simulink model "furuta_rl_balance"  (R2025a)
settings: Solver=VariableStepAuto  StartTime=0.0  StopTime=50  RelTol=1e-3
libraries: rllib x1
settings Model: Creator=deng_zhiwen  LastModifiedBy=deng_zhiwen

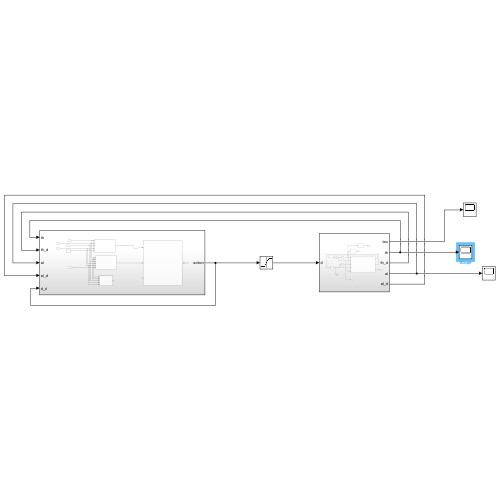
[thumbnail: Simulink's stored preview of the top-level diagram]
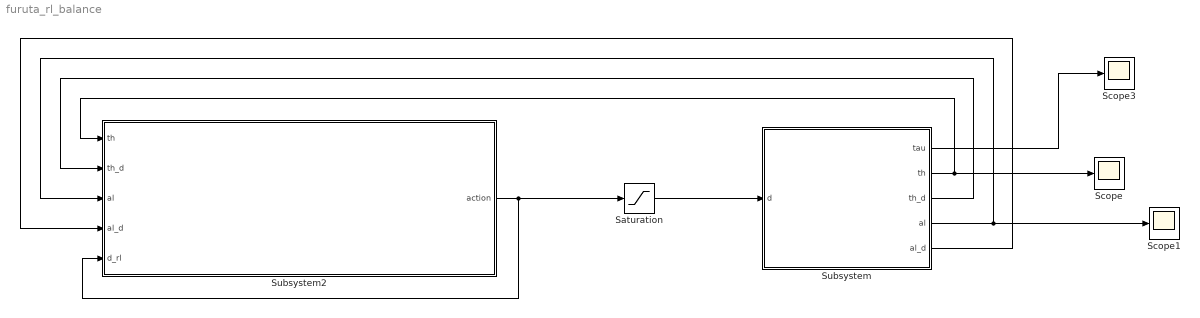
== system furuta_rl_balance ==
  Saturation : Saturate  UpperLimit=1  LowerLimit=-1
  Scope : Scope
      settings: ActiveDisplayYMinimum=-7.2129032176721157  ActiveDisplayYMaximum=4.9641994886210785
  Scope1 : Scope
      settings: ActiveDisplayYMinimum=-7.2858875046268059  ActiveDisplayYMaximum=4.4859787074197675
  Scope3 : Scope
      settings: ActiveDisplayYMinimum=-1  ActiveDisplayYMaximum=1  DataLoggingVariableName=ScopeData3
  Subsystem : Subsystem
  Subsystem2 : Subsystem
  wires:
  Subsystem/2(th) -> Scope/1, Subsystem2/1(th)
  Subsystem/3(th_d) -> Subsystem2/2(th_d)
  Subsystem/4(al) -> Scope1/1, Subsystem2/3(al)
  Subsystem/5(al_d) -> Subsystem2/4(al_d)
  Subsystem2/1(action) -> Saturation/1, Subsystem2/5(d_rl)
  Saturation/1 -> Subsystem/1(d)
  Subsystem/1(tau) -> Scope3/1

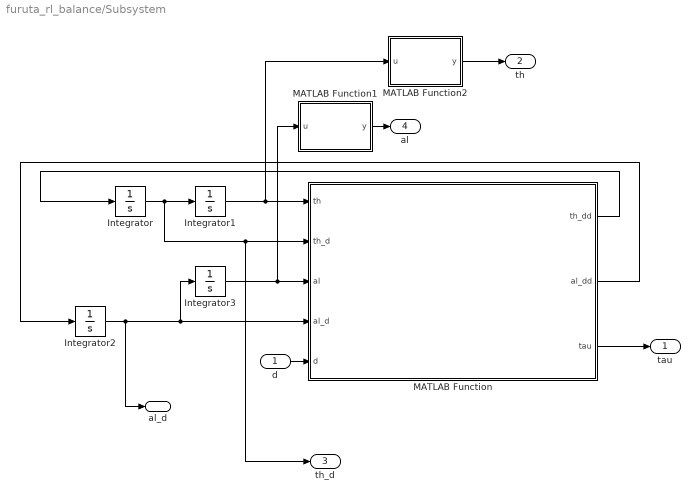
== system furuta_rl_balance/Subsystem ==
  d : Inport
  Integrator : Integrator
  Integrator1 : Integrator
  Integrator2 : Integrator
  Integrator3 : Integrator  InitialCondition=0.3
  MATLAB Function : MATLAB Function  TreatAsAtomicUnit=on
  MATLAB Function1 : MATLAB Function  TreatAsAtomicUnit=on
  MATLAB Function2 : MATLAB Function  TreatAsAtomicUnit=on
  tau : Outport
  th : Outport  Port=2
  th_d : Outport  Port=3
  al : Outport  Port=4
  al_d : Outport  Port=5
  wires:
  MATLAB Function/1(th_dd) -> Integrator/1
  MATLAB Function/2(al_dd) -> Integrator2/1
  Integrator/1 -> Integrator1/1, MATLAB Function/2(th_d), th_d/1
  d/1 -> MATLAB Function/5(d)
  Integrator2/1 -> MATLAB Function/4(al_d), Integrator3/1, al_d/1
  MATLAB Function/3(tau) -> tau/1
  Integrator1/1 -> MATLAB Function2/1(u), MATLAB Function/1(th)
  Integrator3/1 -> MATLAB Function1/1(u), MATLAB Function/3(al)
  MATLAB Function1/1(y) -> al/1
  MATLAB Function2/1(y) -> th/1

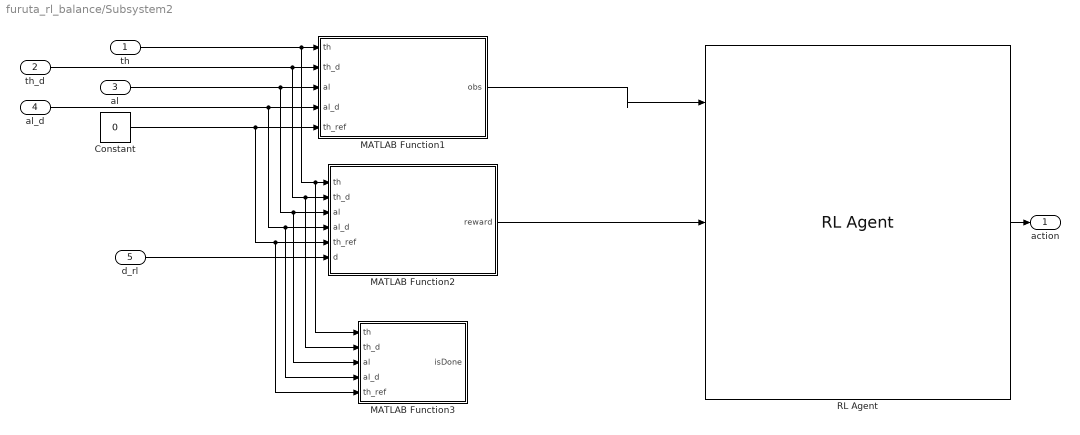
== system furuta_rl_balance/Subsystem2 ==
  th : Inport
  th_d : Inport  Port=2
  al : Inport  Port=3
  al_d : Inport  Port=4
  d_rl : Inport  Port=5
  Constant : Constant  Value=0
  MATLAB Function1 : MATLAB Function  TreatAsAtomicUnit=on
  MATLAB Function2 : MATLAB Function  TreatAsAtomicUnit=on
  MATLAB Function3 : MATLAB Function  TreatAsAtomicUnit=on
  RL Agent : rllib/RL Agent  Agent=agent  ExternalActionAsInput=off  ProvideLastAction=off  ProvideCumRwd=off  TreatAsDirectFeedthrough=on  UseStrictObservationDataTypes=off
  action : Outport
  wires:
  al/1 -> MATLAB Function2/3(al), MATLAB Function3/3(al), MATLAB Function1/3(al)
  th/1 -> MATLAB Function1/1(th), MATLAB Function3/1(th), MATLAB Function2/1(th)
  MATLAB Function2/1(reward) -> RL Agent/2
  MATLAB Function1/1(obs) -> RL Agent/1
  al_d/1 -> MATLAB Function2/4(al_d), MATLAB Function3/4(al_d), MATLAB Function1/4(al_d)
  th_d/1 -> MATLAB Function2/2(th_d), MATLAB Function3/2(th_d), MATLAB Function1/2(th_d)
  d_rl/1 -> MATLAB Function2/6(d)
  RL Agent/1 -> action/1
  Constant/1 -> MATLAB Function2/5(th_ref), MATLAB Function3/5(th_ref), MATLAB Function1/5(th_ref)

== matlab function furuta_rl_balance/Subsystem/MATLAB Function1 ==
  data: u input; y output
function y = wrap_angle(u)
    y = atan2(sin(u), cos(u));
end

== matlab function furuta_rl_balance/Subsystem/MATLAB Function ==
  data: th input; th_dd output; th_d input; al input; al_d input; d input; al_dd output; tau output
function [th_dd, al_dd, tau] = furuta_step(th, th_d, al, al_d, d)
%#codegen
% States: th=theta, th_d=theta_dot, al=alpha, al_d=alpha_dot
% Input:  d = PWM duty [-1, 1]
% Output: th_dd, al_dd [rad/s²], tau [N·m]

% -------------------------------------------------------------------------
% 物理参数
% -------------------------------------------------------------------------
J_theta = 2.5e-4;   % 旋转臂转动惯量        [kg·m²]
J_alpha = 1.2e-3;   % 摆杆转动惯量          [kg·m²]
m_p     = 0.120;    % 摆杆质量              [kg]
r       = 0.1;      % 旋转臂长度            [m]
l       = 0.1;      % 摆杆质心到摆轴距离    [m]
g       = 9.81;     % 重力加速度            [m/s²]
B_r     = 0.0024;   % 旋转臂阻尼系数        [N·m·s/rad]
B_p     = 0.0024;   % 摆轴阻尼系数          [N·m·s/rad]

% 电机参数
K_g     = 9.2767;   % 减速比
V_s     = 5.0;      % 供电电压              [V]
R_m     = 2.5;      % 电枢电阻              [Ω]
k_t     = 0.020;    % 力矩常数              [N·m/A]
k_e     = 0.020;    % 反电动势常数          [V·s/rad]
eta_m   = 0.7;      % 电机效率
eta_g   = 0.7;      % 减速箱效率
tau_max = 0.25;     % 力矩饱和值            [N·m]

% -------------------------------------------------------------------------
% 动力学方程组合参数（从物理参数推导，便于核查）
%
%   惯性矩阵 M = [a,        e*cos(al)]
%               [e*cos(al), c        ]
%
%   a  = J_theta + m_p*r²   旋转臂等效惯量
%   c  = J_alpha + m_p*l²   摆杆等效惯量
%   e  = m_p*r*l            耦合项幅值，实际耦合项 b = e*cos(al)
%   g0 = m_p*g*l            重力项幅值，实际重力项 = g0*sin(al)
% -------------------------------------------------------------------------
a  = J_theta + m_p * r^2;   % = 2.5e-4 + 0.12×0.1² = 1.45e-3  [kg·m²]
c  = J_alpha + m_p * l^2;   % = 1.2e-3 + 0.12×0.1² = 2.40e-3  [kg·m²]
e  = m_p * r * l;           % = 0.12×0.1×0.1        = 1.20e-3  [kg·m²]
g0 = m_p * g * l;           % = 0.12×9.81×0.1       = 0.11772  [N·m]

% -------------------------------------------------------------------------
% 力矩计算: tau = eta_m*eta_g*K_g*k_t*(V_s*d - k_e*K_g*th_d) / R_m
%               = Cd*d - Cv*th_d
% -------------------------------------------------------------------------
Cd = eta_m * eta_g * K_g * k_t * V_s / R_m;       % ≈ 0.18182 [N·m/duty]
Cv = eta_m * eta_g * K_g^2 * k_t * k_e / R_m;     % ≈ 0.00675 [N·m·s/rad]

tau_raw = Cd*d - Cv*th_d;
tau     = max(-tau_max, min(tau_max, tau_raw));     % 力矩饱和
% -------------------------------------------------------------------------
% 构建右端向量
%
%   rhs1 = tau - B_r*th_d + e*sin(al)*al_d²    (θ方程，含离心项)
%   rhs2 =     - B_p*al_d + g0*sin(al)          (α方程，含重力项)
% -------------------------------------------------------------------------
b    = e * cos(al);                        % 惯性矩阵耦合项    [kg·m²]

rhs1 = tau - B_r*th_d + e*sin(al)*al_d^2;
rhs2 =     - B_p*al_d + g0*sin(al);

% -------------------------------------------------------------------------
% 克莱姆法则求解 M*[th_dd; al_dd] = [rhs1; rhs2]
%
%   detM = a*c - b²  (恒 > 0，已验证最小值 a*c-e² = 2.04e-6 > 0)
% -------------------------------------------------------------------------
detM  = a*c - b^2;

th_dd = ( c*rhs1 - b*rhs2) / detM;
al_dd = (-b*rhs1 + a*rhs2) / detM;

end

== matlab function furuta_rl_balance/Subsystem/MATLAB Function2 ==
  data: u input; y output
function y = wrap_angle(u)
    y = atan2(sin(u), cos(u));
end

== matlab function furuta_rl_balance/Subsystem2/MATLAB Function1 ==
  data: th input; obs output; th_d input; al input; al_d input; th_ref input
function obs = obs_builder(th, th_d, al, al_d, th_ref)
%#codegen
% 观测向量构造（推荐版：5维）
%
% obs = [e_th; th_d; cos(al); sin(al); al_d]
%
% 说明：
% 1) e_th = th - th_ref，直接作为位置误差
% 2) 对摆角 al 使用 sin/cos，避免角度表示不连续
% 3) 当前阶段先强调“稳平衡 + 位置误差约束”

e_th = th - th_ref;

obs = zeros(5,1);

% 旋转臂位置误差
obs(1) = e_th;

% 旋转臂角速度
obs(2) = th_d;

% 摆杆姿态
obs(3) = cos(al);
obs(4) = sin(al);

% 摆杆角速度
obs(5) = al_d;

end

== matlab function furuta_rl_balance/Subsystem2/MATLAB Function2 ==
  data: th input; reward output; th_d input; al input; al_d input; th_ref input; d input
function reward = reward_builder(th, th_d, al, al_d, th_ref, d)
%#codegen
% 奖励函数（平滑稳健版）
%
% 目标：
% 1) 保持摆杆 al = 0 附近（倒立）
% 2) 旋转臂 th 跟踪 th_ref
% 3) 抑制速度过大
% 4) 抑制控制输入过大

e_th = th - th_ref;
e_al = wrap_angle(al);

% -----------------------------
% 权重参数（建议先从这组开始）
% -----------------------------
w_al  = 8.0;     % 摆杆角度误差权重（主目标）
w_th  = 1.0;     % 旋转臂位置误差权重
%w_ald = 0.3;     % 摆杆角速度权重
w_ald = 0.8;
%w_thd = 0.05;    % 旋转臂角速度权重
w_thd = 0.15;    % 旋转臂角速度权重
%w_u   = 0.001;   % 控制输入权重
w_u   = 0.003;   % 控制输入权重

% -----------------------------
% 基础奖励
% -----------------------------
reward = 1.0;

% -----------------------------
% 平滑惩罚项
% -----------------------------
reward = reward ...
    - w_al  * (e_al^2) ...
    - w_th  * (e_th^2) ...
    - w_ald * (al_d^2) ...
    - w_thd * (th_d^2) ...
    - w_u   * (d^2);

% -----------------------------
% 小范围稳态奖励
% -----------------------------
if abs(e_al) < 8*pi/180
    reward = reward + 0.5;
end

if abs(e_al) < 5*pi/180 && abs(e_th) < 8*pi/180
    reward = reward + 0.5;
end

if abs(e_al) < 5*pi/180 && abs(al_d) < 0.5 ...
        && abs(e_th) < 8*pi/180 && abs(th_d) < 0.5
    reward = reward + 1.0;
end

% -----------------------------
% 接近失稳时附加惩罚
% -----------------------------
if abs(e_al) > 20*pi/180
    reward = reward - 5.0;
end

end

function y = wrap_angle(u)
y = mod(u + pi, 2*pi) - pi;
end

== matlab function furuta_rl_balance/Subsystem2/MATLAB Function3 ==
  data: th input; isDone output; th_d input; al input; al_d input; th_ref input
function isDone = isdone_builder(th, th_d, al, al_d, th_ref)
%#codegen
% episode终止逻辑
%
% 训练目标：
% 1) 倒立平衡
% 2) 旋转臂不要偏离参考太远
% 3) 速度不要发散

e_th = th - th_ref;
e_al = wrap_angle(al);

isDone = false;

% 1) 摆杆偏离过大：平衡失败
if abs(e_al) > 30*pi/180
    isDone = true;
    return;
end

% 2) 旋转臂偏离参考过大
if abs(e_th) > 0.8
    isDone = true;
    return;
end

% 3) 速度过大：认为系统发散
if abs(al_d) > 20
    isDone = true;
    return;
end

if abs(th_d) > 20
    isDone = true;
    return;
end

end

function y = wrap_angle(u)
y = mod(u + pi, 2*pi) - pi;
end
